simulink model "R2_ELT448_SIMU"  (R2021a)
settings: Solver=VariableStepAuto  StartTime=0.0  StopTime=7/50  RelTol=1e-3
undefined symbols (not defined in the file): D1, Delta
libraries: spsDistributedParametersLineLib x2, spsThreePhaseParallelRLCLoadLib x1, spsThreePhaseTransformerTwoWindingsLib x1, spsThreePhaseVIMeasurementLib x1, spsThreePhaseFaultLib x1, spsThreePhaseSourceLib x1, spspowerguiLib x1
settings Model: Creator=55329  LastModifiedBy=55329

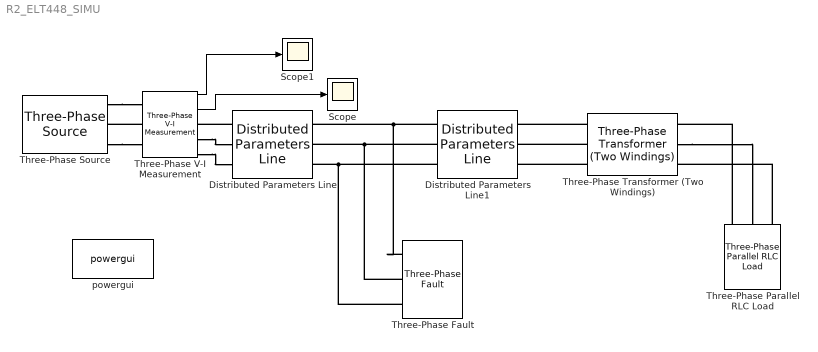
== system R2_ELT448_SIMU ==
  Distributed Parameters Line : spsDistributedParametersLineLib/Distributed Parameters Line  Phases=3  Length=100  Frequency=50  Resistance=[0.01273 0.3864]  Inductance="[0.9337e-3  4.1264e-3]"  Capacitance=[12.74e-9 7.751e-9]  x1=[-0.00058 2.4438818244266e-11 3589.09430489565 -10328.2783447853;-0.00056 2.52133013260996e-11 3653.91751900348 -10305.5236771896;-0.00054 2.59867890299689e-11 3718.59648270417 -10282.362165165;-0.00052 2.67592508199038e-11 3783.12864258297 -10258.7947230883;-0.0005 2.75306562004356e-11 3847.51145102073 -10234.8222813618;-0.00048 2.83009747178006e-11 3911.74236629439 -10210.4457863765;-0.00046 2.90701759611427e-11 3975.8188526774 -10185.6662004746;-0.00044 2.98382295637141e-11 4039.7383805398 -10160.4845019118;-0.00042 3.06051052040735e-11 4103.49842644808 -10134.9016848183;-0.0004 3.13707726072837e-11 4167.0964732648 -10108.9187591601;-0.00038 3.21352015461068e-11 4230.53001024797 -10082.5367506986;-0.00036 3.28983618421971e-11 4293.79653315016 -10055.7567009501;-0.00034 3.3660223367293e-11 4356.89354431738 -10028.5796671454;-0.00032 3.44207560444058e-11 4419.81855278766 -10001.006722187;-0.0003 3.51799298490077e-11 4482.56907438942 -9973.03895460773;-0.00028 3.59377148102169e-11 4545.14263183952 -9944.6774685271;-0.00026 3.66940810119807e-11 4607.53675484103 -9915.92338360804;-0.00024 3.74489985942564e-11 4669.74898018084 -9886.77783501256;-0.00022 3.82024377541905e-11 4731.7768518268 -9857.24197335704;-0.0002 3.89543687472952e-11 4793.61792102474 -9827.31696466671;-0.00018 3.97047618886223e-11 4855.26974639516 -9797.00399032968;-0.00016 4.04535875539355e-11 4916.72989402954 -9766.30424705026;-0.00014 4.12008161808796e-11 4977.99593758649 -9735.21894680177;-0.00012 4.19464182701481e-11 5039.06545838752 -9703.74931677862;-0.0001 4.2690364386647e-11 5099.93604551252 -9671.89659934792;-8e-05 4.34326251606575e-11 5160.60529589493 -9639.66205200042;-6e-05 4.41731712889953e-11 5221.07081441662 -9607.04694730086;-4e-05 4.49119735361672e-11 5281.33021400248 -9574.05257283771;-2e-05 4.56490027355255e-11 5341.38111571456 -9540.68023117239]  x2=[-0.00058 3.2960270768688e-10 3029.77841150658 -10129.185310179;-0.00056 3.49798017269633e-10 3093.36173583232 -10109.9488347897;-0.00054 3.69979517425614e-10 3156.82293953341 -10090.3132359314;-0.00052 3.90146411423754e-10 3220.1595172702 -10070.279288784;-0.0005 4.10297903109608e-10 3283.36896862304 -10049.8477842533;-0.00048 4.3043319693679e-10 3346.44879819102 -10029.0195289402;-0.00046 4.50551497998377e-10 3409.3965156905 -10007.7953451085;-0.00044 4.70652012058291e-10 3472.20963605335 -9986.17607065264;-0.00042 4.90733945582654e-10 3534.88567952515 -9964.16255906462;-0.0004 5.10796505771116e-10 3597.42217176302 -9941.75567940015;-0.00038 5.30838900588154e-10 3659.81664393332 -9918.95631624447;-0.00036 5.50860338794339e-10 3722.06663280912 -9895.76536967739;-0.00034 5.70860029977572e-10 3784.16968086746 -9872.18375523779;-0.00032 5.90837184584291e-10 3846.12333638634 -9848.21240388741;-0.0003 6.10791013950637e-10 3907.92515354151 -9823.85226197417;-0.00028 6.30720730333594e-10 3969.57269250306 -9799.10429119476;-0.00026 6.50625546942085e-10 4031.06351953171 -9773.96946855668;-0.00024 6.70504677968032e-10 4092.3952070749 -9748.4487863397;-0.00022 6.90357338617381e-10 4153.56533386261 -9722.54325205666;-0.0002 7.10182745141082e-10 4214.57148500298 -9696.25388841368;-0.00018 7.29980114866032e-10 4275.41125207763 -9669.58173326984;-0.00016 7.49748666225974e-10 4336.08223323672 -9642.52783959614;-0.00014 7.69487618792348e-10 4396.58203329381 -9615.09327543398;-0.00012 7.89196193305107e-10 4456.90826382038 -9587.27912385299;-0.0001 8.08873611703474e-10 4517.05854324014 -9559.08648290824;-8e-05 8.28519097156664e-10 4577.03049692305 -9530.51646559693;-6e-05 8.48131874094551e-10 4636.82175727908 -9501.5701998144;-4e-05 8.67711168238283e-10 4696.42996385164 -9472.24882830969;-2e-05 8.87256206630852e-10 4755.85276341081 -9442.55350864032]  x3=[-0.00058 -2.08327035865013e-11 17.0951961205475 -19.4164121590465;-0.00056 -2.07780600554123e-11 17.2168547889019 -19.3086173173488;-0.00054 -2.07225962420902e-11 17.3378337653092 -19.200060204501;-0.00052 -2.06663143361512e-11 17.4581282737266 -19.0907451061522;-0.0005 -2.06092165595085e-11 17.5777335651329 -18.9806763378752;-0.00048 -2.05513051662848e-11 17.6966449177159 -18.8698582449964;-0.00046 -2.04925824427225e-11 17.814857637059 -18.7582952024246;-0.00044 -2.04330507070943e-11 17.9323670563266 -18.6459916144774;-0.00042 -2.03727123096112e-11 18.0491685364479 -18.5329519147084;-0.0004 -2.03115696323298e-11 18.1652574663006 -18.4191805657313;-0.00038 -2.02496250890583e-11 18.2806292628923 -18.3046820590442;-0.00036 -2.01868811252612e-11 18.3952793715422 -18.189460914852;-0.00034 -2.01233402179627e-11 18.5092032660603 -18.0735216818882;-0.00032 -2.00590048756491e-11 18.6223964489263 -17.9568689372352;-0.0003 -1.99938776381695e-11 18.7348544514671 -17.8395072861437;-0.00028 -1.99279610766358e-11 18.8465728340334 -17.7214413618507;-0.00026 -1.98612577933209e-11 18.9575471861747 -17.6026758253966;-0.00024 -1.97937704215562e-11 19.0677731268136 -17.4832153654416;-0.00022 -1.97255016256277e-11 19.1772463044187 -17.36306469808;-0.0002 -1.96564541006704e-11 19.2859623971765 -17.2422285666545;-0.00018 -1.95866305725625e-11 19.3939171131616 -17.1207117415686;-0.00016 -1.95160337978173e-11 19.5011061905068 -16.9985190200985;-0.00014 -1.94446665634746e-11 19.6075253975709 -16.8756552262036;-0.00012 -1.93725316869905e-11 19.7131705331057 -16.7521252103361;-0.0001 -1.92996320161265e-11 19.8180374264223 -16.6279338492495;-8e-05 -1.92259704288367e-11 19.9221219375551 -16.5030860458061;-6e-05 -1.91515498331546e-11 20.025419957426 -16.3775867287835;-4e-05 -1.90763731670778e-11 20.127927408006 -16.2514408526798;-2e-05 -1.90004433984523e-11 20.2296402424765 -16.1246533975181]  x4=[-0.00058 2.08864576637608e-11 3.17956297487657 -57.2072052542291;-0.00056 2.08596720980402e-11 3.5389413195051 -57.1860983810558;-0.00054 2.08320630281827e-11 3.89817995278997 -57.1627338986367;-0.00052 2.08036315441471e-11 4.25726469260506 -57.1371127293616;-0.0005 2.07743787683596e-11 4.61618136289968 -57.1092358847103;-0.00048 2.07443058556697e-11 4.97491579425828 -57.079104465213;-0.00046 2.07134139933046e-11 5.33345382445973 -57.0467196604064;-0.00044 2.06817044008221e-11 5.69178129903653 -57.0120827487873;-0.00042 2.06491783300627e-11 6.04988407183353 -56.9751950977617;-0.0004 2.06158370650998e-11 6.40774800556644 -56.9360581635907;-0.00038 2.05816819221895e-11 6.76535897237991 -56.8946734913335;-0.00036 2.05467142497184e-11 7.1227028544053 -56.8510427147862;-0.00034 2.05109354281504e-11 7.47976554431802 -56.8051675564171;-0.00032 2.0474346869972e-11 7.83653294589446 -56.7570498272989;-0.0003 2.04369500196369e-11 8.19299097456849 -56.7066914270372;-0.00028 2.03987463535086e-11 8.54912555798749 -56.6540943436953;-0.00026 2.03597373798026e-11 8.90492263656791 -56.5992606537161;-0.00024 2.03199246385263e-11 9.26036816405031 -56.5421925218397;-0.00022 2.02793097014185e-11 9.61544810805388 -56.4828922010183;-0.0002 2.02378941718875e-11 9.97014845063043 -56.421362032327;-0.00018 2.01956796849474e-11 10.3244551888178 -56.3576044448715;-0.00016 2.01526679071538e-11 10.6783543351926 -56.2916219556923;-0.00014 2.01088605365382e-11 11.0318319184225 -56.2234171696649;-0.00012 2.00642593025405e-11 11.3848739838178 -56.1529927793975;-0.0001 2.0018865965941e-11 11.7374665938822 -56.0803515651246;-8e-05 1.9972682318791e-11 12.0895958288633 -56.0054963945968;-6e-05 1.99257101843417e-11 12.4412477873017 -55.9284302229681;-4e-05 1.98779514169727e-11 12.7924085865804 -55.849156092679;-2e-05 1.98294079021182e-11 13.1430643634721 -55.7676771333364]  x5=0.000565541566995743  V1=ones(3,3)  V2=ones(3,3)  I1=ones(3,3)  I2=ones(3,3)  nHarmo=1  Measurements=None  Decoupling=off  VsMag0=0  VrMag0=0  VsAngle0=0  VrAngle0=0  IsMag0=0  IrMag0=0  IsAngle0=0  IrAngle0=0
      settings: SourceProductBaseCode=PS
  Distributed Parameters Line1 : spsDistributedParametersLineLib/Distributed Parameters Line  Phases=3  Length=100  Frequency=50  Resistance=[0.01273 0.3864]  Inductance="[0.9337e-3  4.1264e-3]"  Capacitance=[12.74e-9 7.751e-9]  x1=[-0.00058 3.2960270768688e-10 3029.77841150658 -10129.185310179;-0.00056 3.49798017269633e-10 3093.36173583232 -10109.9488347897;-0.00054 3.69979517425614e-10 3156.82293953341 -10090.3132359314;-0.00052 3.90146411423754e-10 3220.1595172702 -10070.279288784;-0.0005 4.10297903109608e-10 3283.36896862304 -10049.8477842533;-0.00048 4.3043319693679e-10 3346.44879819102 -10029.0195289402;-0.00046 4.50551497998377e-10 3409.3965156905 -10007.7953451085;-0.00044 4.70652012058291e-10 3472.20963605335 -9986.17607065264;-0.00042 4.90733945582654e-10 3534.88567952515 -9964.16255906462;-0.0004 5.10796505771116e-10 3597.42217176302 -9941.75567940015;-0.00038 5.30838900588154e-10 3659.81664393332 -9918.95631624447;-0.00036 5.50860338794339e-10 3722.06663280912 -9895.76536967739;-0.00034 5.70860029977572e-10 3784.16968086746 -9872.18375523779;-0.00032 5.90837184584291e-10 3846.12333638634 -9848.21240388741;-0.0003 6.10791013950637e-10 3907.92515354151 -9823.85226197417;-0.00028 6.30720730333594e-10 3969.57269250306 -9799.10429119476;-0.00026 6.50625546942085e-10 4031.06351953171 -9773.96946855668;-0.00024 6.70504677968032e-10 4092.3952070749 -9748.4487863397;-0.00022 6.90357338617381e-10 4153.56533386261 -9722.54325205666;-0.0002 7.10182745141082e-10 4214.57148500298 -9696.25388841368;-0.00018 7.29980114866032e-10 4275.41125207763 -9669.58173326984;-0.00016 7.49748666225974e-10 4336.08223323672 -9642.52783959614;-0.00014 7.69487618792348e-10 4396.58203329381 -9615.09327543398;-0.00012 7.89196193305107e-10 4456.90826382038 -9587.27912385299;-0.0001 8.08873611703474e-10 4517.05854324014 -9559.08648290824;-8e-05 8.28519097156664e-10 4577.03049692305 -9530.51646559693;-6e-05 8.48131874094551e-10 4636.82175727908 -9501.5701998144;-4e-05 8.67711168238283e-10 4696.42996385164 -9472.24882830969;-2e-05 8.87256206630852e-10 4755.85276341081 -9442.55350864032]  x2=[-0.00058 3.19649179254825e-10 2440.37811562929 -9809.67293790868;-0.00056 3.40247173042391e-10 2501.96553197851 -9794.14605633241;-0.00054 3.60831734454161e-10 2563.45417501258 -9778.23251864011;-0.00052 3.81402050846897e-10 2624.84161726516 -9761.93295307098;-0.0005 4.01957310139732e-10 2686.12543526513 -9745.24800310398;-0.00048 4.22496700846223e-10 2747.30320963231 -9728.17832743235;-0.00046 4.43019412106394e-10 2808.3725251729 -9710.72459993766;-0.00044 4.63524633718747e-10 2869.33097097491 -9692.88750966319;-0.00042 4.84011556172242e-10 2930.17614050326 -9674.66776078672;-0.0004 5.04479370678259e-10 2990.90563169485 -9656.06607259274;-0.00038 5.24927269202529e-10 3051.51704705336 -9637.08317944405;-0.00036 5.45354444497031e-10 3112.00799374388 -9617.71983075276;-0.00034 5.6576009013186e-10 3172.37608368741 -9597.97679095073;-0.00032 5.86143400527067e-10 3232.61893365514 -9577.85483945936;-0.0003 6.0650357098446e-10 3292.73416536251 -9557.35477065884;-0.00028 6.26839797719371e-10 3352.71940556308 -9536.47739385679;-0.00026 6.47151277892389e-10 3412.5722861423 -9515.22353325629;-0.00024 6.67437209641057e-10 3472.29044421092 -9493.59402792338;-0.00022 6.87696792111523e-10 3531.87152219832 -9471.58973175387;-0.0002 7.07929225490163e-10 3591.31316794556 -9449.21151343972;-0.00018 7.28133711035149e-10 3650.61303479824 -9426.46025643466;-0.00016 7.48309451107988e-10 3709.76878169915 -9403.33685891936;-0.00014 7.68455649205008e-10 3768.7780732807 -9379.84223376596;-0.00012 7.88571509988805e-10 3827.63857995711 -9355.97730850204;-0.0001 8.08656239319638e-10 3886.34797801634 -9331.74302527397;-8e-05 8.28709044286784e-10 3944.9039497119 -9307.14034080977;-6e-05 8.48729133239838e-10 4003.30418335427 -9282.17022638129;-4e-05 8.68715715819969e-10 4061.54637340225 -9256.8336677659;-2e-05 8.8866800299112e-10 4119.62822055388 -9231.13166520754]  x3=[-0.00058 -4.30308982119549e-13 19.1278605787664 -17.3711949711461;-0.00056 -4.03090284428767e-13 19.2366287300321 -17.25066897686;-0.00054 -3.75855673423756e-13 19.344637452134 -17.1294619557005;-0.00052 -3.48606224280326e-13 19.4518824810725 -17.0075786927134;-0.0005 -3.21343012760072e-13 19.5583595829977 -16.8850239996411;-0.00048 -2.940671151679e-13 19.6640645543758 -16.7618027147331;-0.00046 -2.66779608309546e-13 19.7689932221556 -16.6379197025547;-0.00044 -2.39481569449056e-13 19.8731414439329 -16.5133798537952;-0.00042 -2.12174076266261e-13 19.9765051081143 -16.3881880850744;-0.0004 -1.84858206814236e-13 20.0790801340793 -16.2623493387492;-0.00038 -1.57535039476734e-13 20.1808624723415 -16.1358685827176;-0.00036 -1.30205652925616e-13 20.2818481047084 -16.0087508102235;-0.00034 -1.02871126078269e-13 20.3820330444402 -15.8810010396587;-0.00032 -7.55325380550078e-14 20.4814133364071 -15.7526243143655;-0.0003 -4.81909681364767e-14 20.5799850572452 -15.6236257024371;-0.00028 -2.08474957210396e-14 20.6777443155119 -15.494010296518;-0.00026 6.49679971783192e-15 20.774687251839 -15.3637832136024;-0.00024 3.38408386741749e-14 20.8708100390853 -15.2329495948325;-0.00022 6.11835416521519e-14 20.9661088824878 -15.1015146052956;-0.0002 8.85238292086673e-14 21.0605800198114 -14.96948343382;-0.00018 1.15860621995983e-13 21.1542197214973 -14.8368612927703;-0.00016 1.43192840804327e-13 21.2470242908104 -14.7036534178415;-0.00014 1.70519406604501e-13 21.3389900639852 -14.5698650678525;-0.00012 1.97839240590479e-13 21.4301134103705 -14.4355015245382;-0.0001 2.25151264221994e-13 21.5203907325726 -14.3005680923413;-8e-05 2.52454399267117e-13 21.6098184665974 -14.1650700982026;-6e-05 2.79747567844829e-13 21.6983930819911 -14.0290128913508;-4e-05 3.07029692467567e-13 21.7861110819795 -13.8924018430917;-2e-05 3.34299696083765e-13 21.8729690036062 -13.7552423465954]  x4=[-0.00058 4.46674147093937e-13 -2.97771349503067 -57.1139481460807;-0.00056 4.73542430610951e-13 -2.61879955887232 -57.1315301682191;-0.00054 5.0039201948364e-13 -2.25978223699149 -57.1468567353714;-0.00052 5.27221853736208e-13 -1.90067570277731 -57.1599272424708;-0.0005 5.54030874172738e-13 -1.54149413314087 -57.1707411735162;-0.00048 5.80818022419009e-13 -1.18225170795551 -57.179298101592;-0.00046 6.07582240964275e-13 -0.822962609497054 -57.1855976888855;-0.00044 6.34322473203015e-13 -0.463641021883916 -57.1896396866996;-0.00042 6.61037663476647e-13 -0.104301130517114 -57.1914239354632;-0.0004 6.87726757115202e-13 0.25504287847973 -57.1909503647372;-0.00038 7.14388700478964e-13 0.614376818820432 -57.1882189932174;-0.00036 7.4102244100006e-13 0.97368650461631 -57.1832299287338;-0.00034 7.67626927224019e-13 1.33295775093621 -57.1759833682458;-0.00032 7.94201108851279e-13 1.69217637436648 -57.1664795978355;-0.0003 8.20743936778651e-13 2.05132819357097 -57.1547189926953;-0.00028 8.47254363140738e-13 2.41039902985081 -57.1407020171139;-0.00026 8.73731341351301e-13 2.76937470770421 -57.1244292244574;-0.00024 9.00173826144574e-13 3.12824105538609 -57.1059012571478;-0.00022 9.26580773616536e-13 3.4869839054675 -57.0851188466375;-0.0002 9.52951141266116e-13 3.845589095395 -57.0620828133805;-0.00018 9.79283888036352e-13 4.20404246804972 -57.0367940668;-0.00016 1.00557797435549e-12 4.56232987230627 -57.0092536052524;-0.00014 1.03183236217803e-12 4.92043716359143 -56.9794625159879;-0.00012 1.05804601502569e-12 5.2783502044425 -56.9474219751078;-0.0001 1.08421789802834e-12 5.63605486506548 -56.9131332475177;-8e-05 1.11034697796485e-12 5.99353702389287 -56.8765976868778;-6e-05 1.13643222330389e-12 6.35078256814113 -56.8378167355496;-4e-05 1.16247260424464e-12 6.70777739436788 -56.7967919245387;-2e-05 1.18846709275745e-12 7.06450740902865 -56.7535248734342]  x5=0.000565541566995743  V1=ones(3,3)  V2=ones(3,3)  I1=ones(3,3)  I2=ones(3,3)  nHarmo=1  Measurements=None  Decoupling=off  VsMag0=0  VrMag0=0  VsAngle0=0  VrAngle0=0  IsMag0=0  IrMag0=0  IsAngle0=0  IrAngle0=0
      settings: SourceProductBaseCode=PS
  Scope : Scope
  Scope1 : Scope
  Three-Phase Parallel RLC Load : spsThreePhaseParallelRLCLoadLib/Three-Phase Parallel RLC Load  LConnTagsString=A|B|C  Configuration=Y (grounded)  NominalVoltage=0.4e3  Vabc=[1e3 1e3 1e3]  Vabcp=[1e3 1e3 1e3]  NominalFrequency=50  UnbalancedPower=off  ActivePower=10e3  InductivePower=100  CapacitivePower=0  Pabc=[10e3 9e3 11e3]  QLabc=[100 90 110]  QCabc=[100 90 110]  Pabcp=[10e3 9e3 11e3]  QLabcp=[100 90 110]  QCabcp=[100 90 110]  Measurements=None  LoadType=constant Z
  Three-Phase Transformer (Two Windings) : spsThreePhaseTransformerTwoWindingsLib/Three-Phase Transformer (Two Windings)  Winding1Connection=Delta (D1)  Winding2Connection=Yg  CoreType=Three single-phase transformers  SetSaturation=off  Hysteresis=off  DataFile='hysteresis'  SetInitialFlux=off  Measurements=None  UNITS=pu  NominalPower=[ 100e6 , 50 ]  Winding1=[11e3 , 0.002 , 0.08 ]  Winding2=[0.4e3 , 0.002 , 0.08 ]  Rm=500  Lm=500  L0=0.5  Saturation=[ 0,0 ; 0.0024,1.2 ; 1.0,1.52 ]  InitialFluxes=[ 0.8 , -0.8 , 0.7 ]  BreakLoop=off  DiscreteSolver=Trapezoidal iterative  DataType=off  TransfoNumber=1
  Three-Phase V-I Measurement : spsThreePhaseVIMeasurementLib/Three-Phase V-I Measurement  VoltageMeasurement=phase-to-ground  SetLabelV=off  LabelV=Vabc  Vpu=off  VpuLL=off  CurrentMeasurement=yes  SetLabelI=off  LabelI=Iabc  Ipu=off  Pbase=100e6  Vbase=500e3  OutputType=Complex  PhasorSimulation=off  PSBequivalent=0
  Three-Phase Fault : spsThreePhaseFaultLib/Three-Phase Fault  InitialStates=0  FaultA=on  FaultB=on  FaultC=off  GroundFault=off  SwitchTimes="[1/50  5/50]"  External=off  SwitchStatus=NaN  FaultResistance=10000  GroundResistance=0.01  SnubberResistance=1e6  SnubberCapacitance=inf  Measurements=None
  Three-Phase Source : spsThreePhaseSourceLib/Three-Phase Source  InternalConnection=Yg  VoltagePhases=off  Voltage=11e3  PhaseAngle=0  Voltage_phases=[25e3 25e3 25e3]/sqrt(3)  PhaseAngles_phases=[0 -120 +120]  Frequency=50  NonIdealSource=on  SpecifyImpedance=off  Resistance=0.8929  Inductance=16.58e-3  ShortCircuitLevel=100e6  BaseVoltage=11e3  XRratio=7  BusType=swing  Pref=10e3  Qref=0  Prefabc=[10e3, 10e3, 10e3]  Qrefabc=[0, 0, 0]  Qmin=-inf  Qmax=inf
  powergui : spspowerguiLib/powergui  Priority=1  SimulationMode=Discrete  SampleTime=1/50/1000  frequency=60  Iterations=50  frequencyindice=50  Pbase=100e6  ErrMax=1e-4  UnitsV=kV  UnitsW=MW  buscounter=0  FunctionMessages=off  echomessages=off  EnableUseOfTLC=off  CurrentSourceSwitches=off  DisableSnubberDevices=off  DisableRonSwitches=off  DisableVfSwitches=off  DisplayEquations=off  AutomaticDiscreteSolvers=off  SolverType=Tustin/Backward Euler (TBE)  Interpol=off  ExternalGateDelay=off  methode=off  Ts=100  x0status=blocks  SPID=on  SwTol=0  HookPort=off  NonlinearTolerance=1e-4  nMaxIteration=100  ContinueOnMaxIteration=off  RestoreLinks=warning  ResistiveCurrentMeasurement=off  Frange=[0:2:500]  Ylog=off  Xlog=on  ShowGrid=off  save=off  variable=ZData  structure=0  ZoomFFT=off  StartTime=0.0  cycles=1  DisplayStyle=1  fundamental=60  FreqAxis=off  MaxFrequency=1000  frequencyindicesteady=1  RmsSteady=1  display=off
  wires:
  Three-Phase V-I Measurement/2 -> Scope/1
  Three-Phase V-I Measurement/1 -> Scope1/1
  connections:
  Distributed Parameters Line1/LConn1 -- Three-Phase Fault/LConn1 -- Distributed Parameters Line/RConn1
  Distributed Parameters Line1/LConn2 -- Three-Phase Fault/LConn2 -- Distributed Parameters Line/RConn2
  Distributed Parameters Line1/LConn3 -- Three-Phase Fault/LConn3 -- Distributed Parameters Line/RConn3
  Three-Phase Transformer (Two Windings)/LConn1 -- Distributed Parameters Line1/RConn1
  Three-Phase Transformer (Two Windings)/LConn2 -- Distributed Parameters Line1/RConn2
  Three-Phase Transformer (Two Windings)/LConn3 -- Distributed Parameters Line1/RConn3
  Three-Phase Parallel RLC Load/LConn1 -- Three-Phase Transformer (Two Windings)/RConn1
  Three-Phase Transformer (Two Windings)/RConn2 -- Three-Phase Parallel RLC Load/LConn2
  Three-Phase Parallel RLC Load/LConn3 -- Three-Phase Transformer (Two Windings)/RConn3
  Three-Phase V-I Measurement/LConn2 -- Three-Phase Source/RConn2
  Three-Phase Source/RConn1 -- Three-Phase V-I Measurement/LConn1
  Three-Phase Source/RConn3 -- Three-Phase V-I Measurement/LConn3
  Distributed Parameters Line/LConn1 -- Three-Phase V-I Measurement/RConn1
  Three-Phase V-I Measurement/RConn2 -- Distributed Parameters Line/LConn2
  Three-Phase V-I Measurement/RConn3 -- Distributed Parameters Line/LConn3
